simulink library "actuator_T2_lib"  (Simulink 6.6)
undefined symbols (not defined in the file or in its folder): bias
libraries: aeroutilslib x18, simulink x1
settings Model: Creator=amurch  LastModifiedBy=amurch

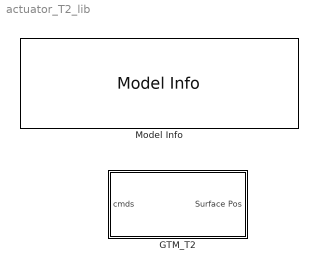
== system actuator_T2_lib ==
  GTM_T2 : Subsystem
  Model Info : simulink/Model-Wide Utilities/Model Info  SystemSampleTime=-1  InitialBlockCM=None  BlockCM=None  Frame=on  DisplayStringWithTags=|  HorizontalTextAlignment=Center  LeftAlignmentValue=0.5  SourceBlockDiagram=actuator_T2_lib  TagMaxNumber=20
      | Actuator Library
      | %<ModelVersion>
      | Las modified by %<LastModifiedBy> on %<LastModificationDate>

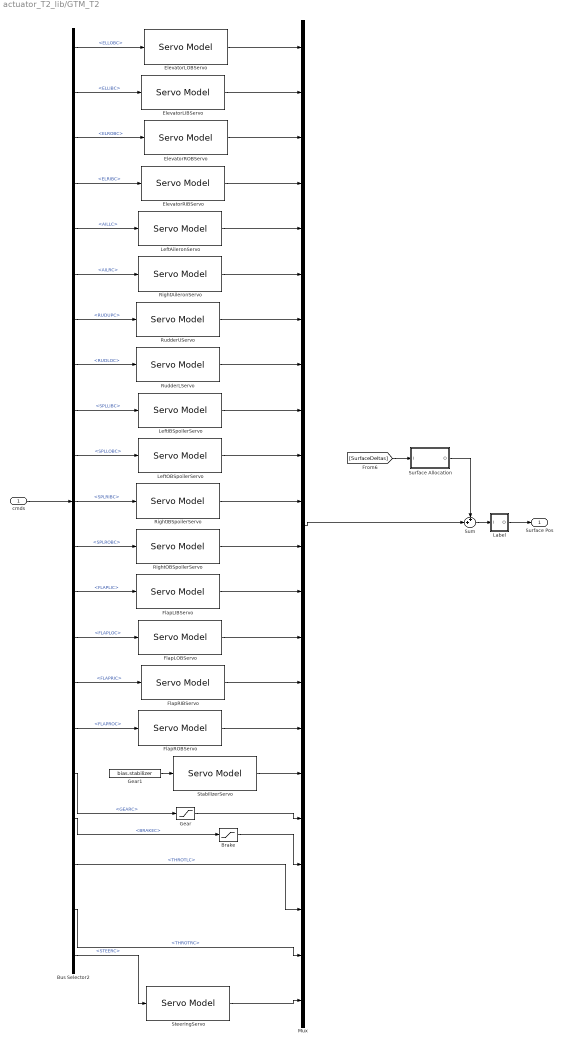
== system actuator_T2_lib/GTM_T2 ==
  cmds : Inport
  Brake : Saturate  UpperLimit=1.0  LowerLimit=0.0
  Bus Selector2 : BusSelector  OutputSignals=ELLOBC,ELLIBC,ELROBC,ELRIBC,AILLC,AILRC,RUDUPC,RUDLOC,SPLLIBC,SPLLOBC,SPLRIBC,SPLROBC,FLAPLIC,FLAPLOC,FLAPRIC,FLAPROC,GEARC,BRAKEC,THROTLC,THROTRC,STEERC
  ElevatorLIBServo : aeroutilslib/Servo Model  SystemSampleTime=-1  freq=10  RL=300  POS_hi=20  POS_lo=-30
  ElevatorLOBServo : aeroutilslib/Servo Model  SystemSampleTime=-1  freq=10  RL=300  POS_hi=20  POS_lo=-30
  ElevatorRIBServo : aeroutilslib/Servo Model  SystemSampleTime=-1  freq=10  RL=300  POS_hi=20  POS_lo=-30
  ElevatorROBServo : aeroutilslib/Servo Model  SystemSampleTime=-1  freq=10  RL=300  POS_hi=20  POS_lo=-30
  FlapLIBServo : aeroutilslib/Servo Model  SystemSampleTime=-1  freq=10  RL=300  POS_hi=30  POS_lo=0
  FlapLOBServo : aeroutilslib/Servo Model  SystemSampleTime=-1  freq=10  RL=300  POS_hi=30  POS_lo=0
  FlapRIBServo : aeroutilslib/Servo Model  SystemSampleTime=-1  freq=10  RL=300  POS_hi=30  POS_lo=0
  FlapROBServo : aeroutilslib/Servo Model  SystemSampleTime=-1  freq=10  RL=300  POS_hi=30  POS_lo=0
  Gear : Saturate  UpperLimit=1.0  LowerLimit=0.0
  Gear1 : Constant  Value=bias.stabilizer
  Label : Subsystem
  LeftAileronServo : aeroutilslib/Servo Model  SystemSampleTime=-1  freq=10  RL=300  POS_hi=20.0  POS_lo=-20
  LeftIBSpoilerServo : aeroutilslib/Servo Model  SystemSampleTime=-1  freq=10  RL=300  POS_hi=15  POS_lo=0
  LeftOBSpoilerServo : aeroutilslib/Servo Model  SystemSampleTime=-1  freq=10  RL=300  POS_hi=45  POS_lo=0
  Mux : Mux  Inputs=22
  RightAileronServo : aeroutilslib/Servo Model  SystemSampleTime=-1  freq=10  RL=300  POS_hi=20.0  POS_lo=-20
  RightIBSpoilerServo : aeroutilslib/Servo Model  SystemSampleTime=-1  freq=10  RL=300  POS_hi=15  POS_lo=0
  RightOBSpoilerServo : aeroutilslib/Servo Model  SystemSampleTime=-1  freq=10  RL=300  POS_hi=45  POS_lo=0
  RudderLServo : aeroutilslib/Servo Model  SystemSampleTime=-1  freq=8.43  RL=300  POS_hi=30  POS_lo=-30.0
  RudderUServo : aeroutilslib/Servo Model  SystemSampleTime=-1  freq=8.43  RL=300  POS_hi=30  POS_lo=-30.0
  StabilizerServo : aeroutilslib/Servo Model  SystemSampleTime=-1  freq=10  RL=300  POS_hi=4  POS_lo=-12
  SteeringServo : aeroutilslib/Servo Model  SystemSampleTime=-1  freq=10  RL=300  POS_hi=30  POS_lo=0
  Sum : Sum  Inputs=++|
  Surface Allocation : Subsystem
  Surface Pos : Outport
  wires:
  Sum/1 -> Label/1(I)
  Label/1(O) -> Surface Pos/1
  [SurfaceDeltas] -> Surface Allocation/1(I)
  Bus Selector2/13 -> FlapLIBServo/1  "<FLAPLIC>"
  Bus Selector2/14 -> FlapLOBServo/1  "<FLAPLOC>"
  Bus Selector2/15 -> FlapRIBServo/1  "<FLAPRIC>"
  Bus Selector2/16 -> FlapROBServo/1  "<FLAPROC>"
  Bus Selector2/17 -> Gear/1  "<GEARC>"
  Bus Selector2/18 -> Brake/1  "<BRAKEC>"
  Mux/1 -> Sum/2
  Bus Selector2/1 -> ElevatorLOBServo/1  "<ELLOBC>"
  Bus Selector2/2 -> ElevatorLIBServo/1  "<ELLIBC>"
  ElevatorLOBServo/1 -> Mux/1
  ElevatorLIBServo/1 -> Mux/2
  Bus Selector2/3 -> ElevatorROBServo/1  "<ELROBC>"
  ElevatorROBServo/1 -> Mux/3
  Bus Selector2/4 -> ElevatorRIBServo/1  "<ELRIBC>"
  ElevatorRIBServo/1 -> Mux/4
  Bus Selector2/5 -> LeftAileronServo/1  "<AILLC>"
  LeftAileronServo/1 -> Mux/5
  Bus Selector2/6 -> RightAileronServo/1  "<AILRC>"
  RightAileronServo/1 -> Mux/6
  RudderUServo/1 -> Mux/7
  Bus Selector2/7 -> RudderUServo/1  "<RUDUPC>"
  Bus Selector2/8 -> RudderLServo/1  "<RUDLOC>"
  Bus Selector2/9 -> LeftIBSpoilerServo/1  "<SPLLIBC>"
  Bus Selector2/10 -> LeftOBSpoilerServo/1  "<SPLLOBC>"
  Bus Selector2/11 -> RightIBSpoilerServo/1  "<SPLRIBC>"
  Bus Selector2/12 -> RightOBSpoilerServo/1  "<SPLROBC>"
  RudderLServo/1 -> Mux/8
  LeftIBSpoilerServo/1 -> Mux/9
  LeftOBSpoilerServo/1 -> Mux/10
  RightIBSpoilerServo/1 -> Mux/11
  RightOBSpoilerServo/1 -> Mux/12
  FlapLIBServo/1 -> Mux/13
  FlapLOBServo/1 -> Mux/14
  FlapRIBServo/1 -> Mux/15
  FlapROBServo/1 -> Mux/16
  StabilizerServo/1 -> Mux/17
  Gear/1 -> Mux/18
  Brake/1 -> Mux/19
  cmds/1 -> Bus Selector2/1
  Surface Allocation/1(O) -> Sum/1
  Gear1/1 -> StabilizerServo/1
  Bus Selector2/19 -> Mux/20  "<THROTLC>"
  Bus Selector2/20 -> Mux/21  "<THROTRC>"
  Bus Selector2/21 -> SteeringServo/1  "<STEERC>"
  SteeringServo/1 -> Mux/22

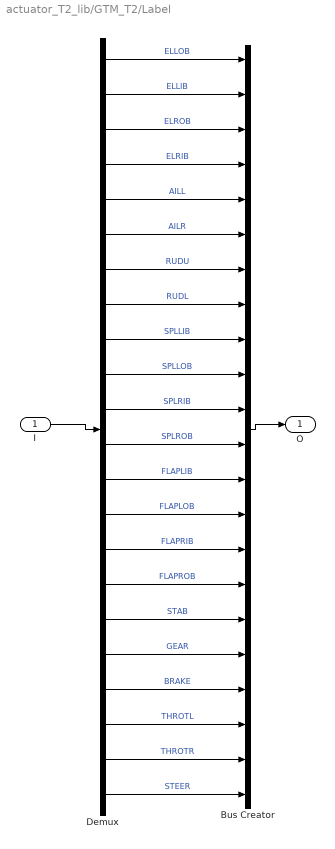
== system actuator_T2_lib/GTM_T2/Label ==
  I : Inport
  Bus Creator : BusCreator  Inputs=22
  Demux : Demux  Outputs=22
  O : Outport
  wires:
  I/1 -> Demux/1
  Bus Creator/1 -> O/1
  Demux/2 -> Bus Creator/2  "ELLIB"
  Demux/3 -> Bus Creator/3  "ELROB"
  Demux/4 -> Bus Creator/4  "ELRIB"
  Demux/5 -> Bus Creator/5  "AILL"
  Demux/6 -> Bus Creator/6  "AILR"
  Demux/7 -> Bus Creator/7  "RUDU"
  Demux/8 -> Bus Creator/8  "RUDL"
  Demux/9 -> Bus Creator/9  "SPLLIB"
  Demux/10 -> Bus Creator/10  "SPLLOB"
  Demux/11 -> Bus Creator/11  "SPLRIB"
  Demux/12 -> Bus Creator/12  "SPLROB"
  Demux/13 -> Bus Creator/13  "FLAPLIB"
  Demux/14 -> Bus Creator/14  "FLAPLOB"
  Demux/15 -> Bus Creator/15  "FLAPRIB"
  Demux/16 -> Bus Creator/16  "FLAPROB"
  Demux/17 -> Bus Creator/17  "STAB"
  Demux/18 -> Bus Creator/18  "GEAR"
  Demux/1 -> Bus Creator/1  "ELLOB"
  Demux/19 -> Bus Creator/19  "BRAKE"
  Demux/20 -> Bus Creator/20  "THROTL"
  Demux/21 -> Bus Creator/21  "THROTR"
  Demux/22 -> Bus Creator/22  "STEER"

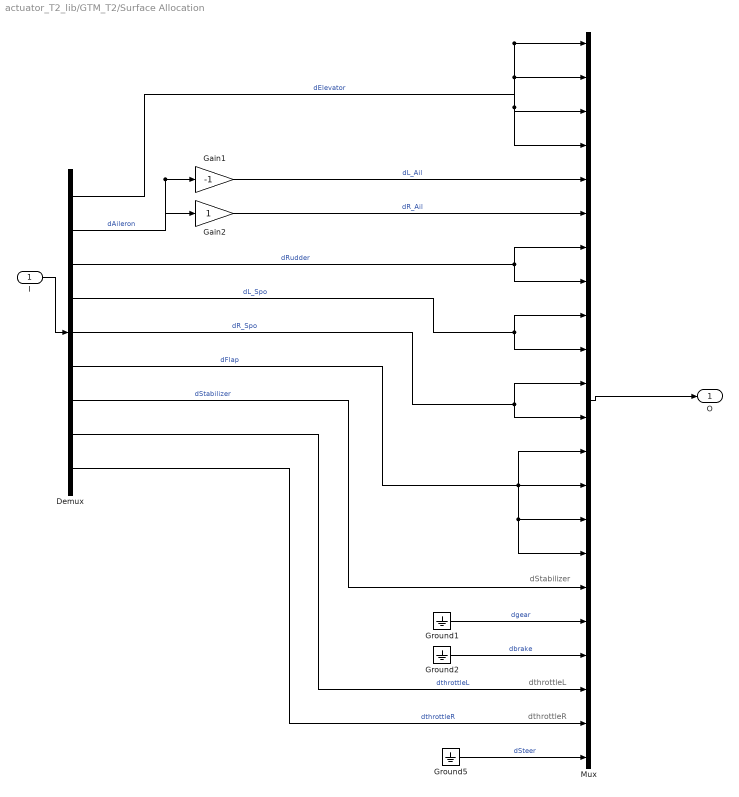
== system actuator_T2_lib/GTM_T2/Surface Allocation ==
  note: dthrottleR
  note: dthrottleL
  note: dStabilizer
  I : Inport
  Demux : Demux  Outputs=9
  Gain1 : Gain  Gain=-1
  Gain2 : Gain
  Ground1 : Ground
  Ground2 : Ground
  Ground5 : Ground
  Mux : Mux  Inputs=22
  O : Outport
  wires:
  I/1 -> Demux/1
  Gain1/1 -> Mux/5  "dL_Ail"
  Gain2/1 -> Mux/6  "dR_Ail"
  Mux/1 -> O/1
  Ground1/1 -> Mux/18  "dgear"
  Ground2/1 -> Mux/19  "dbrake"
  Ground5/1 -> Mux/22  "dSteer"
  Demux/3 -> Mux/7, Mux/8  "dRudder"
  Demux/8 -> Mux/20  "dthrottleL"
  Demux/9 -> Mux/21  "dthrottleR"
  Demux/2 -> Gain1/1, Gain2/1  "dAileron"
  Demux/1 -> Mux/1, Mux/2, Mux/3, Mux/4  "dElevator"
  Demux/4 -> Mux/9, Mux/10  "dL_Spo"
  Demux/5 -> Mux/11, Mux/12  "dR_Spo"
  Demux/6 -> Mux/14, Mux/13, Mux/15, Mux/16  "dFlap"
  Demux/7 -> Mux/17  "dStabilizer"
